simulink model "simulation_3d"  (R2023b)
settings: Solver=ode4  StartTime=0.0  StopTime=2  FixedStep=0.001  RelTol=1e-3  EnableMultiTasking=on
values from neighbouring files (symbols this model uses):
  compKd = 1    [main.m]
  compKi = 0    [main.m]
  compKp = 1    [main.m]
  derivative_filter_samples = 1    [parameters.m]
  gain = 0.00285714285714    [paper_data.mat]    (also in parameters.m = 0.025)
  initial_q = q    [main.m]    (also in paper_data.mat = [0 0 0 0.2 0 0.2]; stuff.mat = [0 0 0 0 0 0])
  initial_states = [tau(1), tau(2), q_dot(1), q_dot(2), q_dot(3), q_dot(4),                     q_dot(5), q_dot(6),q(1), q(2), q(3), q(4), q(5), q(6),                     x_ICR, v(1), v(2), bld_ang(1), bld_ang(2), bld_ang(3)]    [main.m]    (also in paper_data.mat = [56000 56000 0 0 0 0 0 0 0 0 0 0.2 ... (20 elements, 1x20)]; stuff.mat = [56000 56000 0 0 0 0 0 0 0 0 0 0 ... (20 elements, 20x1)])
  initial_v = v    [main.m]    (also in paper_data.mat = [0 0]; stuff.mat = [0 0])
  L = 1.4    [paper_data.mat]    (also in parameters.m = 1.2; stuff.mat)
  l = 2.349    [paper_data.mat]    (also in parameters.m; stuff.mat; test.m = vd_parmas(3))
  stop_distance = 0.3    [paper_data.mat]    (also in parameters.m)
  type = 0.9    [paper_data.mat]    (also in parameters.m; stuff.mat = 0.2)
  v_limit = [velocity_limit, turn_vel_limit]    [main.m]
undefined symbols (not defined in the file or in its folder): DiscIntNeverNeededParam
libraries: fuzblock x10, slpidlib x6, simulink x2
settings Model: Creator=frog  LastModifiedBy=srd2
settings SolverCC: AlgebraicLoopSolver=TrustRegion
settings DataIOCC: ExternalInput=[in]  InitialState=pathlength
settings DebuggingCC: UnconnectedInputMsg=warning  UnconnectedOutputMsg=warning  UnconnectedLineMsg=warning  UnderSpecifiedDimensionMsg=warning
settings ModelReferenceCC: EnableRefExpFcnMdlSchedulingChecks=on
settings RTWCC: DLArmComputeVersion=19.05

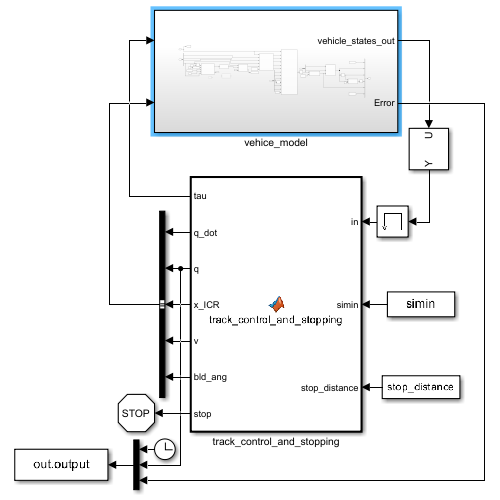
[thumbnail: Simulink's stored preview of the top-level diagram]
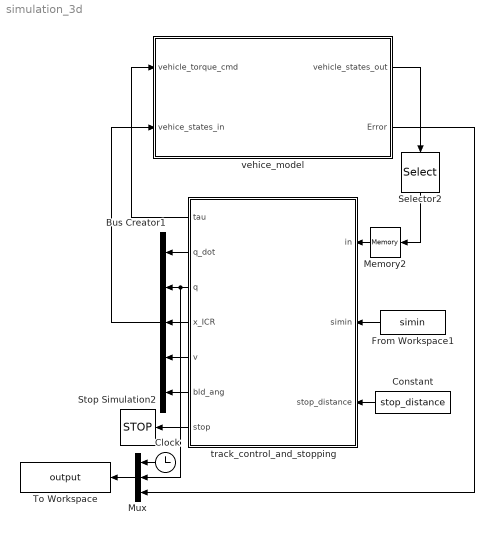
== system simulation_3d ==
  Bus Creator1 : BusCreator  Inputs=5
  Clock : Clock
  Constant : Constant  Value=stop_distance
  From Workspace1 : FromWorkspace  VariableName=simin
  Memory2 : Memory  InitialCondition=initial_states  InheritSampleTime=on
  Mux : Mux  Inputs=3
  Selector2 : Selector  InputPortWidth=20  IndexOptions=Index vector (dialog)  Indices=[1 2 3 4 5 6 7 8 9 10 11 12 13 14 15 16 17 18 19 20]  OutputSizes=1
  Stop Simulation2 : Stop
  To Workspace : ToWorkspace  VariableName=output  SaveFormat=Timeseries  SampleTime=-1
  track_control_and_stopping : MATLAB Function  TreatAsAtomicUnit=on
  vehice_model : Subsystem
  wires:
  Bus Creator1/1 -> vehice_model/2(vehice_states_in)
  vehice_model/1(vehicle_states_out) -> Selector2/1
  track_control_and_stopping/7(stop) -> Stop Simulation2/1
  From Workspace1/1 -> track_control_and_stopping/2(simin)
  Selector2/1 -> Memory2/1
  Memory2/1 -> track_control_and_stopping/1(in)
  track_control_and_stopping/5(v) -> Bus Creator1/4
  track_control_and_stopping/4(x_ICR) -> Bus Creator1/3
  track_control_and_stopping/3(q) -> Bus Creator1/2, Mux/2
  track_control_and_stopping/1(tau) -> vehice_model/1(vehicle_torque_cmd)
  track_control_and_stopping/6(bld_ang) -> Bus Creator1/5
  Mux/1 -> To Workspace/1
  Clock/1 -> Mux/1
  vehice_model/2(Error) -> Mux/3
  Constant/1 -> track_control_and_stopping/3(stop_distance)
  track_control_and_stopping/2(q_dot) -> Bus Creator1/1

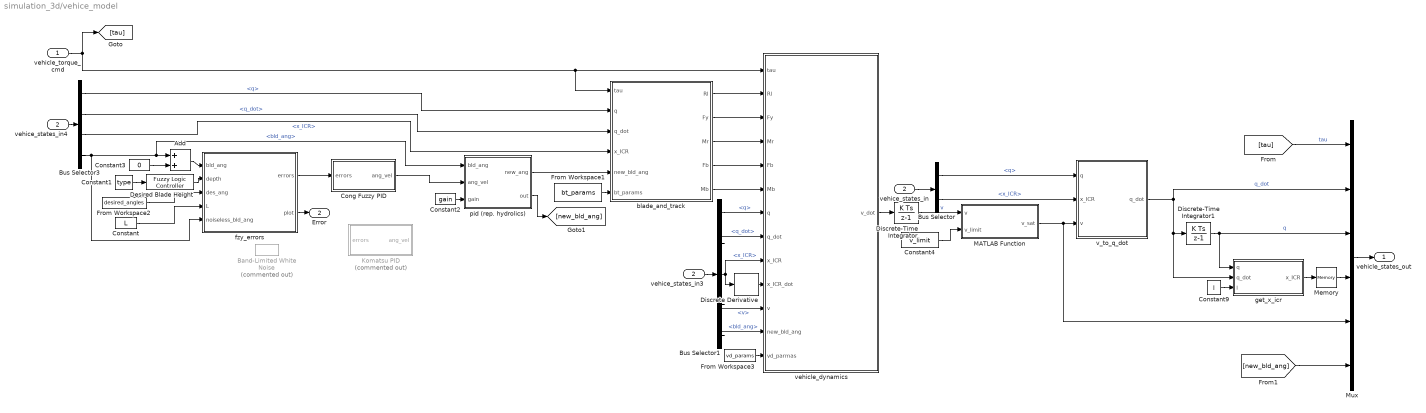
== system simulation_3d/vehice_model ==
  vehicle_torque_cmd : Inport
  vehice_states_in : Inport  Port=2
  Add : Sum
  Band-Limited White Noise : simulink/Sources/Band-Limited White Noise  Commented=on  Cov=[1e-4]  Ts=0.0001  seed=[23341]
  Bus Selector : BusSelector  OutputSignals=q,x_ICR
  Bus Selector1 : BusSelector  OutputSignals=q,q_dot,x_ICR,v,bld_ang
  Bus Selector3 : BusSelector  OutputSignals=q,q_dot,x_ICR,bld_ang
  Cong Fuzzy PID : Subsystem
  Constant : Constant  Value=L
  Constant1 : Constant  Value=type
  Constant2 : Constant  Value=gain
  Constant3 : Constant  Value=0
  Constant4 : Constant  Value=v_limit
  Constant9 : Constant  Value=l
  Desired Blade Height : fuzblock/Fuzzy Logic  Controller  FIS='blade_height.fis'  OutputSampleNumber=101  DataType=double  FuzzifiedInputs=off  RuleFiringStrengths=off  RuleOutputs=off  AggregatedOutputs=off  SimulateUsing=Interpreted execution  OutOfRangeInputValueMessage=warning  NoRuleFiredMessage=warning  EmptyOutputFuzzySetMessage=warning
  Discrete Derivative : simulink/Discrete/Discrete Derivative  gainval=1.0  ICPrevScaledInput=0.0  OutMin=[]  OutMax=[]  OutDataType=fixdt(1, 16)  OutScaling=2^-10  DoSatur=off
  Discrete-Time Integrator : DiscreteIntegrator  InitialCondition=initial_v  SampleTime=-1  ICPrevOutput=DiscIntNeverNeededParam  ICPrevScaledInput=DiscIntNeverNeededParam
  Discrete-Time Integrator1 : DiscreteIntegrator  InitialCondition=initial_q  SampleTime=-1  ICPrevOutput=DiscIntNeverNeededParam  ICPrevScaledInput=DiscIntNeverNeededParam
  From Workspace1 : FromWorkspace  VariableName=bt_params
  From Workspace2 : FromWorkspace  VariableName=desired_angles
  From Workspace3 : FromWorkspace  VariableName=vd_params
  Komatsu PID : Subsystem  Commented=on
  MATLAB Function : MATLAB Function  TreatAsAtomicUnit=on
  Memory : Memory  InheritSampleTime=on  LinearizeAsDelay=on
  Mux : Mux  Inputs=6
  blade_and_track : MATLAB Function  TreatAsAtomicUnit=on
  fzy_errors : MATLAB Function  TreatAsAtomicUnit=on
  get_x_icr : MATLAB Function  TreatAsAtomicUnit=on
  pid (rep. hydrolics) : MATLAB Function  TreatAsAtomicUnit=on
  v_to_q_dot : MATLAB Function  TreatAsAtomicUnit=on
  vehice_states_in3 : InportShadow  Port=2
  vehice_states_in4 : InportShadow  Port=2
  vehicle_dynamics : MATLAB Function  TreatAsAtomicUnit=on
  vehicle_states_out : Outport
  Error : Outport  Port=2
  wires:
  Mux/1 -> vehicle_states_out/1
  Discrete-Time Integrator1/1 -> Mux/3, get_x_icr/1(q)  "q"
  v_to_q_dot/1(q_dot) -> Mux/2, Discrete-Time Integrator1/1, get_x_icr/2(q_dot)  "q_dot"
  vehice_states_in/1 -> Bus Selector/1
  vehicle_dynamics/1(v_dot) -> Discrete-Time Integrator/1
  [tau] -> Mux/1  "tau"
  blade_and_track/3(Mr) -> vehicle_dynamics/4(Mr)
  blade_and_track/2(Fy) -> vehicle_dynamics/3(Fy)
  blade_and_track/1(Rl) -> vehicle_dynamics/2(Rl)
  vehice_states_in3/1 -> Bus Selector1/1
  Bus Selector1/2 -> vehicle_dynamics/8(q_dot)  "<q_dot>"
  vehicle_torque_cmd/1 -> blade_and_track/1(tau), vehicle_dynamics/1(tau), [tau]
  Bus Selector3/1 -> blade_and_track/2(q)  "<q>"
  Bus Selector3/2 -> blade_and_track/3(q_dot)  "<q_dot>"
  Bus Selector3/3 -> blade_and_track/4(x_ICR)  "<x_ICR>"
  Bus Selector1/4 -> vehicle_dynamics/11(v)  "<v>"
  Bus Selector/1 -> v_to_q_dot/1(q)  "<q>"
  Bus Selector1/1 -> vehicle_dynamics/7(q)  "<q>"
  Discrete Derivative/1 -> vehicle_dynamics/10(x_ICR_dot)
  Bus Selector1/3 -> vehicle_dynamics/9(x_ICR), Discrete Derivative/1  "<x_ICR>"
  Bus Selector/2 -> v_to_q_dot/2(x_ICR)  "<x_ICR>"
  vehice_states_in4/1 -> Bus Selector3/1
  get_x_icr/1(x_ICR) -> Memory/1
  blade_and_track/4(Fb) -> vehicle_dynamics/5(Fb)
  Desired Blade Height/1 -> fzy_errors/2(depth)
  Bus Selector1/5 -> vehicle_dynamics/12(new_bld_ang)  "<bld_ang>"
  blade_and_track/5(Mb) -> vehicle_dynamics/6(Mb)
  Constant1/1 -> Desired Blade Height/1
  Bus Selector3/4 -> pid (rep. hydrolics)/1(bld_ang), Add/1, fzy_errors/5(noiseless_bld_ang)  "<bld_ang>"
  pid (rep. hydrolics)/1(new_ang) -> blade_and_track/5(new_bld_ang)
  [new_bld_ang] -> Mux/6
  pid (rep. hydrolics)/2(out) -> [new_bld_ang]
  Constant9/1 -> get_x_icr/3(l)
  From Workspace2/1 -> fzy_errors/3(des_ang)
  From Workspace1/1 -> blade_and_track/6(bt_params)
  From Workspace3/1 -> vehicle_dynamics/13(vd_parmas)
  fzy_errors/2(plot) -> Error/1
  Constant/1 -> fzy_errors/4(L)
  Constant2/1 -> pid (rep. hydrolics)/3(gain)
  Memory/1 -> Mux/4
  Add/1 -> fzy_errors/1(bld_ang)
  Constant3/1 -> Add/2
  Constant4/1 -> MATLAB Function/2(v_limit)
  Discrete-Time Integrator/1 -> MATLAB Function/1(v)  "v"
  MATLAB Function/1(v_sat) -> v_to_q_dot/3(v), Mux/5
  fzy_errors/1(errors) -> Cong Fuzzy PID/1(errors)
  Cong Fuzzy PID/1(ang_vel) -> pid (rep. hydrolics)/2(ang_vel)

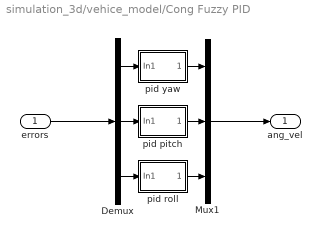
== system simulation_3d/vehice_model/Cong Fuzzy PID ==
  errors : Inport
  Demux : Demux  Outputs=3
  Mux1 : Mux  Inputs=3
  pid pitch : Subsystem
  pid roll : Subsystem
  pid yaw : Subsystem
  ang_vel : Outport
  wires:
  Demux/2 -> pid pitch/1(In1)
  pid yaw/1(Out1) -> Mux1/1
  Demux/3 -> pid roll/1(In1)
  pid roll/1(Out1) -> Mux1/3
  pid pitch/1(Out1) -> Mux1/2
  Demux/1 -> pid yaw/1(In1)
  errors/1 -> Demux/1
  Mux1/1 -> ang_vel/1

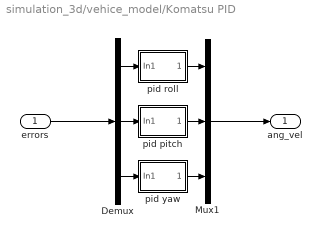
== system simulation_3d/vehice_model/Komatsu PID ==
  errors : Inport
  Demux : Demux  Outputs=3
  Mux1 : Mux  Inputs=3
  pid pitch : Subsystem
  pid roll : Subsystem
  pid yaw : Subsystem
  ang_vel : Outport
  wires:
  Demux/2 -> pid pitch/1(In1)
  pid roll/1(Out1) -> Mux1/1
  Demux/3 -> pid yaw/1(In1)
  pid yaw/1(Out1) -> Mux1/3
  pid pitch/1(Out1) -> Mux1/2
  Demux/1 -> pid roll/1(In1)
  errors/1 -> Demux/1
  Mux1/1 -> ang_vel/1

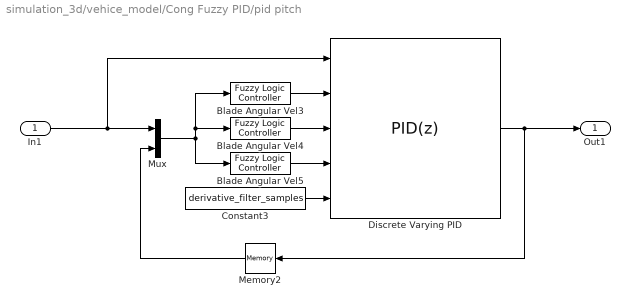
== system simulation_3d/vehice_model/Cong Fuzzy PID/pid pitch ==
  In1 : Inport
  Blade Angular Vel3 : fuzblock/Fuzzy Logic  Controller  FIS='comparision_Kp.fis'  OutputSampleNumber=101  DataType=double  FuzzifiedInputs=off  RuleFiringStrengths=off  RuleOutputs=off  AggregatedOutputs=off  SimulateUsing=Interpreted execution  OutOfRangeInputValueMessage=warning  NoRuleFiredMessage=warning  EmptyOutputFuzzySetMessage=warning
  Blade Angular Vel4 : fuzblock/Fuzzy Logic  Controller  FIS='comparision_Ki.fis'  OutputSampleNumber=101  DataType=double  FuzzifiedInputs=off  RuleFiringStrengths=off  RuleOutputs=off  AggregatedOutputs=off  SimulateUsing=Interpreted execution  OutOfRangeInputValueMessage=warning  NoRuleFiredMessage=warning  EmptyOutputFuzzySetMessage=warning
  Blade Angular Vel5 : fuzblock/Fuzzy Logic  Controller  FIS='comparision_Kd.fis'  OutputSampleNumber=101  DataType=double  FuzzifiedInputs=off  RuleFiringStrengths=off  RuleOutputs=off  AggregatedOutputs=off  SimulateUsing=Interpreted execution  OutOfRangeInputValueMessage=warning  NoRuleFiredMessage=warning  EmptyOutputFuzzySetMessage=warning
  Constant3 : Constant  Value=derivative_filter_samples
  Discrete Varying PID : slpidlib/PID Controller  Controller=PID  Form=Parallel  TimeDomain=Discrete-time  UseExternalTs=off  SampleTime=-1  IntegratorMethod=Forward Euler  FilterMethod=Forward Euler  ControllerParametersSource=external  P=1  I=1  UseKiTs=off  D=0  N=100  UseFilter=on  TunerSelectOption=Transfer Function Based (PID Tuner App)  InitialConditionSource=internal  InitialConditionForIntegrator=0  InitialConditionForFilter=0  DifferentiatorICPrevScaledInput=0  ExternalReset=none  TrackingMode=off  Kt=1  LimitOutput=off  SatLimitsSource=internal  UpperSaturationLimit=inf  LowerSaturationLimit=-inf  LinearizeAsGain=on  AntiWindupMode=none  Kb=1  LimitIntegrator=off  UpperIntegratorSaturationLimit=inf  LowerIntegratorSaturationLimit=-inf  POutMin=[]  POutMax=[]  IOutMin=[]  IOutMax=[]  DOutMin=[]  DOutMax=[]  NOutMin=[]  NOutMax=[]  SumOutMin=[]  SumOutMax=[]  SaturationOutMin=[]  SaturationOutMax=[]  PParamMin=[]  PParamMax=[]  IParamMin=[]  IParamMax=[]  DParamMin=[]  DParamMax=[]  NParamMin=[]  NParamMax=[]  KbParamMin=[]  KbParamMax=[]  KtParamMin=[]  KtParamMax=[]  KbOutMin=[]  KbOutMax=[]  KtOutMin=[]  KtOutMax=[]  IntegratorOutMin=[]  IntegratorOutMax=[]  FilterOutMin=[]  FilterOutMax=[]  SumI1OutMin=[]  SumI1OutMax=[]  SumI2OutMin=[]  SumI2OutMax=[]  SumI3OutMin=[]  SumI3OutMax=[]  SumI4OutMin=[]  SumI4OutMax=[]  SumDOutMin=[]  SumDOutMax=[]  DifferentiatorOutMin=[]  DifferentiatorOutMax=[]  FilterDiffOutCoefMin=[]  FilterDiffOutCoefMax=[]  ReciprocalOutMin=[]  ReciprocalOutMax=[]  SumDenOutMin=[]  SumDenOutMax=[]  SumNumOutMin=[]  SumNumOutMax=[]  DivideOutMin=[]  DivideOutMax=[]  UdiffTsProdOutMin=[]  UdiffTsProdOutMax=[]  NTsProdOutMin=[]  NTsProdOutMax=[]  UintegralTsProdOutMin=[]  UintegralTsProdOutMax=[]  UngainTsProdOutMin=[]  UngainTsProdOutMax=[]  ClampingZeroOutDataTypeStr=Inherit: Inherit via back propagation  ClampingZeroOutMin=[]  ClampingZeroOutMax=[]  FilterDenConstantOutDataTypeStr=Inherit: Inherit via back propagation  FilterDenConstantOutMin=[]  FilterDenConstantOutMax=[]  PCopyOutDataTypeStr=Inherit: Inherit via back propagation  PCopyOutMin=[]  PCopyOutMax=[]  NCopyOutDataTypeStr=Inherit: Inherit via back propagation  NCopyOutMin=[]  NCopyOutMax=[]  IntegratorContinuousStateAttributes=''  IntegratorStateMustResolveToSignalObject=off  IntegratorRTWStateStorageClass=Auto  FilterContinuousStateAttributes=''  FilterStateMustResolveToSignalObject=off  FilterRTWStateStorageClass=Auto  ParallelPVariant=ExternalParameters  IdealPVariant=Disabled  IVariant=ExternalParameters  DVariant=ExternalParameters  IntegratorVariant=Discrete  SatVariant=Disabled  AWVariant=Passthrough  PCopyVariant=Disabled  TRVariant=Disabled  FdbkBlocksVariant=Forward  IdealPFdbkVariant=Disabled  SatFdbkVariant=Disabled  DerivativeFilterVariant=ForwardEulerFilter  NVariant=ExternalParameters  NCopyVariant=Disabled  FilterICVariant=InternalICsFilter  IntegratorICVariant=InternalICs  ExternalResetVariant=Disabled  TRSumVariant=Passthrough  SumFdbkVariant=Disabled  SumVariant=Sum_PID  TsampFilterVariant=InternalTs  TsampNgainVariant=Passthrough  TsampIntegralVariant=Disabled_SignalSpec  ExternalSaturationOutDataTypeStr=Inherit: Same as second input
      settings: LibrarySourceBlock=cstblocks/Linear Parameter Varying/Discrete Varying PID
  Memory2 : Memory  InheritSampleTime=on  LinearizeAsDelay=on
  Mux : Mux  Inputs=2
  Out1 : Outport
  wires:
  Blade Angular Vel5/1 -> Discrete Varying PID/4
  Discrete Varying PID/1 -> Memory2/1, Out1/1
  Constant3/1 -> Discrete Varying PID/5
  Blade Angular Vel3/1 -> Discrete Varying PID/2
  Blade Angular Vel4/1 -> Discrete Varying PID/3
  In1/1 -> Mux/1, Discrete Varying PID/1
  Memory2/1 -> Mux/2
  Mux/1 -> Blade Angular Vel5/1, Blade Angular Vel4/1, Blade Angular Vel3/1

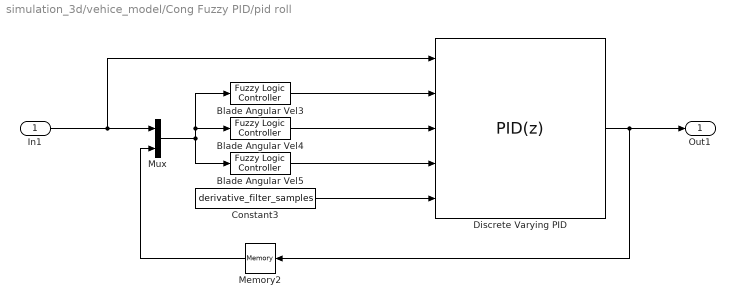
== system simulation_3d/vehice_model/Cong Fuzzy PID/pid roll ==
  In1 : Inport
  Blade Angular Vel3 : fuzblock/Fuzzy Logic  Controller  FIS='comparision_Kp.fis'  OutputSampleNumber=101  DataType=double  FuzzifiedInputs=off  RuleFiringStrengths=off  RuleOutputs=off  AggregatedOutputs=off  SimulateUsing=Interpreted execution  OutOfRangeInputValueMessage=warning  NoRuleFiredMessage=warning  EmptyOutputFuzzySetMessage=warning
  Blade Angular Vel4 : fuzblock/Fuzzy Logic  Controller  FIS='comparision_Ki.fis'  OutputSampleNumber=101  DataType=double  FuzzifiedInputs=off  RuleFiringStrengths=off  RuleOutputs=off  AggregatedOutputs=off  SimulateUsing=Interpreted execution  OutOfRangeInputValueMessage=warning  NoRuleFiredMessage=warning  EmptyOutputFuzzySetMessage=warning
  Blade Angular Vel5 : fuzblock/Fuzzy Logic  Controller  FIS='comparision_Kd.fis'  OutputSampleNumber=101  DataType=double  FuzzifiedInputs=off  RuleFiringStrengths=off  RuleOutputs=off  AggregatedOutputs=off  SimulateUsing=Interpreted execution  OutOfRangeInputValueMessage=warning  NoRuleFiredMessage=warning  EmptyOutputFuzzySetMessage=warning
  Constant3 : Constant  Value=derivative_filter_samples
  Discrete Varying PID : slpidlib/PID Controller  Controller=PID  Form=Parallel  TimeDomain=Discrete-time  UseExternalTs=off  SampleTime=-1  IntegratorMethod=Forward Euler  FilterMethod=Forward Euler  ControllerParametersSource=external  P=1  I=1  UseKiTs=off  D=0  N=100  UseFilter=on  TunerSelectOption=Transfer Function Based (PID Tuner App)  InitialConditionSource=internal  InitialConditionForIntegrator=0  InitialConditionForFilter=0  DifferentiatorICPrevScaledInput=0  ExternalReset=none  TrackingMode=off  Kt=1  LimitOutput=off  SatLimitsSource=internal  UpperSaturationLimit=inf  LowerSaturationLimit=-inf  LinearizeAsGain=on  AntiWindupMode=none  Kb=1  LimitIntegrator=off  UpperIntegratorSaturationLimit=inf  LowerIntegratorSaturationLimit=-inf  POutMin=[]  POutMax=[]  IOutMin=[]  IOutMax=[]  DOutMin=[]  DOutMax=[]  NOutMin=[]  NOutMax=[]  SumOutMin=[]  SumOutMax=[]  SaturationOutMin=[]  SaturationOutMax=[]  PParamMin=[]  PParamMax=[]  IParamMin=[]  IParamMax=[]  DParamMin=[]  DParamMax=[]  NParamMin=[]  NParamMax=[]  KbParamMin=[]  KbParamMax=[]  KtParamMin=[]  KtParamMax=[]  KbOutMin=[]  KbOutMax=[]  KtOutMin=[]  KtOutMax=[]  IntegratorOutMin=[]  IntegratorOutMax=[]  FilterOutMin=[]  FilterOutMax=[]  SumI1OutMin=[]  SumI1OutMax=[]  SumI2OutMin=[]  SumI2OutMax=[]  SumI3OutMin=[]  SumI3OutMax=[]  SumI4OutMin=[]  SumI4OutMax=[]  SumDOutMin=[]  SumDOutMax=[]  DifferentiatorOutMin=[]  DifferentiatorOutMax=[]  FilterDiffOutCoefMin=[]  FilterDiffOutCoefMax=[]  ReciprocalOutMin=[]  ReciprocalOutMax=[]  SumDenOutMin=[]  SumDenOutMax=[]  SumNumOutMin=[]  SumNumOutMax=[]  DivideOutMin=[]  DivideOutMax=[]  UdiffTsProdOutMin=[]  UdiffTsProdOutMax=[]  NTsProdOutMin=[]  NTsProdOutMax=[]  UintegralTsProdOutMin=[]  UintegralTsProdOutMax=[]  UngainTsProdOutMin=[]  UngainTsProdOutMax=[]  ClampingZeroOutDataTypeStr=Inherit: Inherit via back propagation  ClampingZeroOutMin=[]  ClampingZeroOutMax=[]  FilterDenConstantOutDataTypeStr=Inherit: Inherit via back propagation  FilterDenConstantOutMin=[]  FilterDenConstantOutMax=[]  PCopyOutDataTypeStr=Inherit: Inherit via back propagation  PCopyOutMin=[]  PCopyOutMax=[]  NCopyOutDataTypeStr=Inherit: Inherit via back propagation  NCopyOutMin=[]  NCopyOutMax=[]  IntegratorContinuousStateAttributes=''  IntegratorStateMustResolveToSignalObject=off  IntegratorRTWStateStorageClass=Auto  FilterContinuousStateAttributes=''  FilterStateMustResolveToSignalObject=off  FilterRTWStateStorageClass=Auto  ParallelPVariant=ExternalParameters  IdealPVariant=Disabled  IVariant=ExternalParameters  DVariant=ExternalParameters  IntegratorVariant=Discrete  SatVariant=Disabled  AWVariant=Passthrough  PCopyVariant=Disabled  TRVariant=Disabled  FdbkBlocksVariant=Forward  IdealPFdbkVariant=Disabled  SatFdbkVariant=Disabled  DerivativeFilterVariant=ForwardEulerFilter  NVariant=ExternalParameters  NCopyVariant=Disabled  FilterICVariant=InternalICsFilter  IntegratorICVariant=InternalICs  ExternalResetVariant=Disabled  TRSumVariant=Passthrough  SumFdbkVariant=Disabled  SumVariant=Sum_PID  TsampFilterVariant=InternalTs  TsampNgainVariant=Passthrough  TsampIntegralVariant=Disabled_SignalSpec  ExternalSaturationOutDataTypeStr=Inherit: Same as second input
      settings: LibrarySourceBlock=cstblocks/Linear Parameter Varying/Discrete Varying PID
  Memory2 : Memory  InheritSampleTime=on  LinearizeAsDelay=on
  Mux : Mux  Inputs=2
  Out1 : Outport
  wires:
  Blade Angular Vel5/1 -> Discrete Varying PID/4
  Discrete Varying PID/1 -> Memory2/1, Out1/1
  Constant3/1 -> Discrete Varying PID/5
  Blade Angular Vel3/1 -> Discrete Varying PID/2
  Blade Angular Vel4/1 -> Discrete Varying PID/3
  In1/1 -> Mux/1, Discrete Varying PID/1
  Memory2/1 -> Mux/2
  Mux/1 -> Blade Angular Vel5/1, Blade Angular Vel4/1, Blade Angular Vel3/1

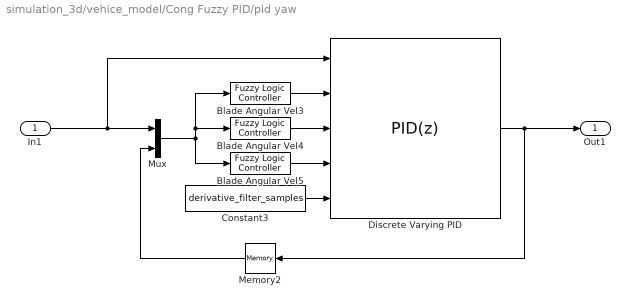
== system simulation_3d/vehice_model/Cong Fuzzy PID/pid yaw ==
  In1 : Inport
  Blade Angular Vel3 : fuzblock/Fuzzy Logic  Controller  FIS='comparision_Kp.fis'  OutputSampleNumber=101  DataType=double  FuzzifiedInputs=off  RuleFiringStrengths=off  RuleOutputs=off  AggregatedOutputs=off  SimulateUsing=Interpreted execution  OutOfRangeInputValueMessage=warning  NoRuleFiredMessage=warning  EmptyOutputFuzzySetMessage=warning
  Blade Angular Vel4 : fuzblock/Fuzzy Logic  Controller  FIS='comparision_Ki.fis'  OutputSampleNumber=101  DataType=double  FuzzifiedInputs=off  RuleFiringStrengths=off  RuleOutputs=off  AggregatedOutputs=off  SimulateUsing=Interpreted execution  OutOfRangeInputValueMessage=warning  NoRuleFiredMessage=warning  EmptyOutputFuzzySetMessage=warning
  Blade Angular Vel5 : fuzblock/Fuzzy Logic  Controller  FIS='comparision_Kd.fis'  OutputSampleNumber=101  DataType=double  FuzzifiedInputs=off  RuleFiringStrengths=off  RuleOutputs=off  AggregatedOutputs=off  SimulateUsing=Interpreted execution  OutOfRangeInputValueMessage=warning  NoRuleFiredMessage=warning  EmptyOutputFuzzySetMessage=warning
  Constant3 : Constant  Value=derivative_filter_samples
  Discrete Varying PID : slpidlib/PID Controller  Controller=PID  Form=Parallel  TimeDomain=Discrete-time  UseExternalTs=off  SampleTime=-1  IntegratorMethod=Forward Euler  FilterMethod=Forward Euler  ControllerParametersSource=external  P=1  I=1  UseKiTs=off  D=0  N=100  UseFilter=on  TunerSelectOption=Transfer Function Based (PID Tuner App)  InitialConditionSource=internal  InitialConditionForIntegrator=0  InitialConditionForFilter=0  DifferentiatorICPrevScaledInput=0  ExternalReset=none  TrackingMode=off  Kt=1  LimitOutput=off  SatLimitsSource=internal  UpperSaturationLimit=inf  LowerSaturationLimit=-inf  LinearizeAsGain=on  AntiWindupMode=none  Kb=1  LimitIntegrator=off  UpperIntegratorSaturationLimit=inf  LowerIntegratorSaturationLimit=-inf  POutMin=[]  POutMax=[]  IOutMin=[]  IOutMax=[]  DOutMin=[]  DOutMax=[]  NOutMin=[]  NOutMax=[]  SumOutMin=[]  SumOutMax=[]  SaturationOutMin=[]  SaturationOutMax=[]  PParamMin=[]  PParamMax=[]  IParamMin=[]  IParamMax=[]  DParamMin=[]  DParamMax=[]  NParamMin=[]  NParamMax=[]  KbParamMin=[]  KbParamMax=[]  KtParamMin=[]  KtParamMax=[]  KbOutMin=[]  KbOutMax=[]  KtOutMin=[]  KtOutMax=[]  IntegratorOutMin=[]  IntegratorOutMax=[]  FilterOutMin=[]  FilterOutMax=[]  SumI1OutMin=[]  SumI1OutMax=[]  SumI2OutMin=[]  SumI2OutMax=[]  SumI3OutMin=[]  SumI3OutMax=[]  SumI4OutMin=[]  SumI4OutMax=[]  SumDOutMin=[]  SumDOutMax=[]  DifferentiatorOutMin=[]  DifferentiatorOutMax=[]  FilterDiffOutCoefMin=[]  FilterDiffOutCoefMax=[]  ReciprocalOutMin=[]  ReciprocalOutMax=[]  SumDenOutMin=[]  SumDenOutMax=[]  SumNumOutMin=[]  SumNumOutMax=[]  DivideOutMin=[]  DivideOutMax=[]  UdiffTsProdOutMin=[]  UdiffTsProdOutMax=[]  NTsProdOutMin=[]  NTsProdOutMax=[]  UintegralTsProdOutMin=[]  UintegralTsProdOutMax=[]  UngainTsProdOutMin=[]  UngainTsProdOutMax=[]  ClampingZeroOutDataTypeStr=Inherit: Inherit via back propagation  ClampingZeroOutMin=[]  ClampingZeroOutMax=[]  FilterDenConstantOutDataTypeStr=Inherit: Inherit via back propagation  FilterDenConstantOutMin=[]  FilterDenConstantOutMax=[]  PCopyOutDataTypeStr=Inherit: Inherit via back propagation  PCopyOutMin=[]  PCopyOutMax=[]  NCopyOutDataTypeStr=Inherit: Inherit via back propagation  NCopyOutMin=[]  NCopyOutMax=[]  IntegratorContinuousStateAttributes=''  IntegratorStateMustResolveToSignalObject=off  IntegratorRTWStateStorageClass=Auto  FilterContinuousStateAttributes=''  FilterStateMustResolveToSignalObject=off  FilterRTWStateStorageClass=Auto  ParallelPVariant=ExternalParameters  IdealPVariant=Disabled  IVariant=ExternalParameters  DVariant=ExternalParameters  IntegratorVariant=Discrete  SatVariant=Disabled  AWVariant=Passthrough  PCopyVariant=Disabled  TRVariant=Disabled  FdbkBlocksVariant=Forward  IdealPFdbkVariant=Disabled  SatFdbkVariant=Disabled  DerivativeFilterVariant=ForwardEulerFilter  NVariant=ExternalParameters  NCopyVariant=Disabled  FilterICVariant=InternalICsFilter  IntegratorICVariant=InternalICs  ExternalResetVariant=Disabled  TRSumVariant=Passthrough  SumFdbkVariant=Disabled  SumVariant=Sum_PID  TsampFilterVariant=InternalTs  TsampNgainVariant=Passthrough  TsampIntegralVariant=Disabled_SignalSpec  ExternalSaturationOutDataTypeStr=Inherit: Same as second input
      settings: LibrarySourceBlock=cstblocks/Linear Parameter Varying/Discrete Varying PID
  Memory2 : Memory  InheritSampleTime=on  LinearizeAsDelay=on
  Mux : Mux  Inputs=2
  Out1 : Outport
  wires:
  Blade Angular Vel5/1 -> Discrete Varying PID/4
  Discrete Varying PID/1 -> Memory2/1, Out1/1
  Constant3/1 -> Discrete Varying PID/5
  Blade Angular Vel3/1 -> Discrete Varying PID/2
  Blade Angular Vel4/1 -> Discrete Varying PID/3
  In1/1 -> Mux/1, Discrete Varying PID/1
  Memory2/1 -> Mux/2
  Mux/1 -> Blade Angular Vel5/1, Blade Angular Vel4/1, Blade Angular Vel3/1

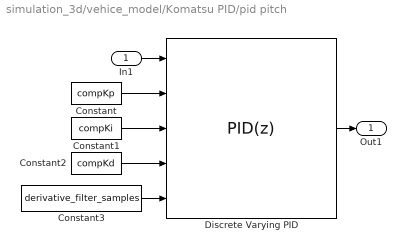
== system simulation_3d/vehice_model/Komatsu PID/pid pitch ==
  In1 : Inport
  Constant : Constant  Value=compKp
  Constant1 : Constant  Value=compKi
  Constant2 : Constant  Value=compKd
  Constant3 : Constant  Value=derivative_filter_samples
  Discrete Varying PID : slpidlib/PID Controller  Controller=PID  Form=Parallel  TimeDomain=Discrete-time  UseExternalTs=off  SampleTime=-1  IntegratorMethod=Forward Euler  FilterMethod=Forward Euler  ControllerParametersSource=external  P=1  I=1  UseKiTs=off  D=0  N=100  UseFilter=on  TunerSelectOption=Transfer Function Based (PID Tuner App)  InitialConditionSource=internal  InitialConditionForIntegrator=0  InitialConditionForFilter=0  DifferentiatorICPrevScaledInput=0  ExternalReset=none  TrackingMode=off  Kt=1  LimitOutput=off  SatLimitsSource=internal  UpperSaturationLimit=inf  LowerSaturationLimit=-inf  LinearizeAsGain=on  AntiWindupMode=none  Kb=1  LimitIntegrator=off  UpperIntegratorSaturationLimit=inf  LowerIntegratorSaturationLimit=-inf  POutMin=[]  POutMax=[]  IOutMin=[]  IOutMax=[]  DOutMin=[]  DOutMax=[]  NOutMin=[]  NOutMax=[]  SumOutMin=[]  SumOutMax=[]  SaturationOutMin=[]  SaturationOutMax=[]  PParamMin=[]  PParamMax=[]  IParamMin=[]  IParamMax=[]  DParamMin=[]  DParamMax=[]  NParamMin=[]  NParamMax=[]  KbParamMin=[]  KbParamMax=[]  KtParamMin=[]  KtParamMax=[]  KbOutMin=[]  KbOutMax=[]  KtOutMin=[]  KtOutMax=[]  IntegratorOutMin=[]  IntegratorOutMax=[]  FilterOutMin=[]  FilterOutMax=[]  SumI1OutMin=[]  SumI1OutMax=[]  SumI2OutMin=[]  SumI2OutMax=[]  SumI3OutMin=[]  SumI3OutMax=[]  SumI4OutMin=[]  SumI4OutMax=[]  SumDOutMin=[]  SumDOutMax=[]  DifferentiatorOutMin=[]  DifferentiatorOutMax=[]  FilterDiffOutCoefMin=[]  FilterDiffOutCoefMax=[]  ReciprocalOutMin=[]  ReciprocalOutMax=[]  SumDenOutMin=[]  SumDenOutMax=[]  SumNumOutMin=[]  SumNumOutMax=[]  DivideOutMin=[]  DivideOutMax=[]  UdiffTsProdOutMin=[]  UdiffTsProdOutMax=[]  NTsProdOutMin=[]  NTsProdOutMax=[]  UintegralTsProdOutMin=[]  UintegralTsProdOutMax=[]  UngainTsProdOutMin=[]  UngainTsProdOutMax=[]  ClampingZeroOutDataTypeStr=Inherit: Inherit via back propagation  ClampingZeroOutMin=[]  ClampingZeroOutMax=[]  FilterDenConstantOutDataTypeStr=Inherit: Inherit via back propagation  FilterDenConstantOutMin=[]  FilterDenConstantOutMax=[]  PCopyOutDataTypeStr=Inherit: Inherit via back propagation  PCopyOutMin=[]  PCopyOutMax=[]  NCopyOutDataTypeStr=Inherit: Inherit via back propagation  NCopyOutMin=[]  NCopyOutMax=[]  IntegratorContinuousStateAttributes=''  IntegratorStateMustResolveToSignalObject=off  IntegratorRTWStateStorageClass=Auto  FilterContinuousStateAttributes=''  FilterStateMustResolveToSignalObject=off  FilterRTWStateStorageClass=Auto  ParallelPVariant=ExternalParameters  IdealPVariant=Disabled  IVariant=ExternalParameters  DVariant=ExternalParameters  IntegratorVariant=Discrete  SatVariant=Disabled  AWVariant=Passthrough  PCopyVariant=Disabled  TRVariant=Disabled  FdbkBlocksVariant=Forward  IdealPFdbkVariant=Disabled  SatFdbkVariant=Disabled  DerivativeFilterVariant=ForwardEulerFilter  NVariant=ExternalParameters  NCopyVariant=Disabled  FilterICVariant=InternalICsFilter  IntegratorICVariant=InternalICs  ExternalResetVariant=Disabled  TRSumVariant=Passthrough  SumFdbkVariant=Disabled  SumVariant=Sum_PID  TsampFilterVariant=InternalTs  TsampNgainVariant=Passthrough  TsampIntegralVariant=Disabled_SignalSpec  ExternalSaturationOutDataTypeStr=Inherit: Same as second input
      settings: LibrarySourceBlock=cstblocks/Linear Parameter Varying/Discrete Varying PID
  Out1 : Outport
  wires:
  Constant2/1 -> Discrete Varying PID/4
  Discrete Varying PID/1 -> Out1/1
  Constant3/1 -> Discrete Varying PID/5
  Constant/1 -> Discrete Varying PID/2
  Constant1/1 -> Discrete Varying PID/3
  In1/1 -> Discrete Varying PID/1

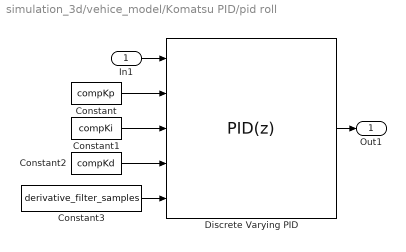
== system simulation_3d/vehice_model/Komatsu PID/pid roll ==
  In1 : Inport
  Constant : Constant  Value=compKp
  Constant1 : Constant  Value=compKi
  Constant2 : Constant  Value=compKd
  Constant3 : Constant  Value=derivative_filter_samples
  Discrete Varying PID : slpidlib/PID Controller  Controller=PID  Form=Parallel  TimeDomain=Discrete-time  UseExternalTs=off  SampleTime=-1  IntegratorMethod=Forward Euler  FilterMethod=Forward Euler  ControllerParametersSource=external  P=1  I=1  UseKiTs=off  D=0  N=100  UseFilter=on  TunerSelectOption=Transfer Function Based (PID Tuner App)  InitialConditionSource=internal  InitialConditionForIntegrator=0  InitialConditionForFilter=0  DifferentiatorICPrevScaledInput=0  ExternalReset=none  TrackingMode=off  Kt=1  LimitOutput=off  SatLimitsSource=internal  UpperSaturationLimit=inf  LowerSaturationLimit=-inf  LinearizeAsGain=on  AntiWindupMode=none  Kb=1  LimitIntegrator=off  UpperIntegratorSaturationLimit=inf  LowerIntegratorSaturationLimit=-inf  POutMin=[]  POutMax=[]  IOutMin=[]  IOutMax=[]  DOutMin=[]  DOutMax=[]  NOutMin=[]  NOutMax=[]  SumOutMin=[]  SumOutMax=[]  SaturationOutMin=[]  SaturationOutMax=[]  PParamMin=[]  PParamMax=[]  IParamMin=[]  IParamMax=[]  DParamMin=[]  DParamMax=[]  NParamMin=[]  NParamMax=[]  KbParamMin=[]  KbParamMax=[]  KtParamMin=[]  KtParamMax=[]  KbOutMin=[]  KbOutMax=[]  KtOutMin=[]  KtOutMax=[]  IntegratorOutMin=[]  IntegratorOutMax=[]  FilterOutMin=[]  FilterOutMax=[]  SumI1OutMin=[]  SumI1OutMax=[]  SumI2OutMin=[]  SumI2OutMax=[]  SumI3OutMin=[]  SumI3OutMax=[]  SumI4OutMin=[]  SumI4OutMax=[]  SumDOutMin=[]  SumDOutMax=[]  DifferentiatorOutMin=[]  DifferentiatorOutMax=[]  FilterDiffOutCoefMin=[]  FilterDiffOutCoefMax=[]  ReciprocalOutMin=[]  ReciprocalOutMax=[]  SumDenOutMin=[]  SumDenOutMax=[]  SumNumOutMin=[]  SumNumOutMax=[]  DivideOutMin=[]  DivideOutMax=[]  UdiffTsProdOutMin=[]  UdiffTsProdOutMax=[]  NTsProdOutMin=[]  NTsProdOutMax=[]  UintegralTsProdOutMin=[]  UintegralTsProdOutMax=[]  UngainTsProdOutMin=[]  UngainTsProdOutMax=[]  ClampingZeroOutDataTypeStr=Inherit: Inherit via back propagation  ClampingZeroOutMin=[]  ClampingZeroOutMax=[]  FilterDenConstantOutDataTypeStr=Inherit: Inherit via back propagation  FilterDenConstantOutMin=[]  FilterDenConstantOutMax=[]  PCopyOutDataTypeStr=Inherit: Inherit via back propagation  PCopyOutMin=[]  PCopyOutMax=[]  NCopyOutDataTypeStr=Inherit: Inherit via back propagation  NCopyOutMin=[]  NCopyOutMax=[]  IntegratorContinuousStateAttributes=''  IntegratorStateMustResolveToSignalObject=off  IntegratorRTWStateStorageClass=Auto  FilterContinuousStateAttributes=''  FilterStateMustResolveToSignalObject=off  FilterRTWStateStorageClass=Auto  ParallelPVariant=ExternalParameters  IdealPVariant=Disabled  IVariant=ExternalParameters  DVariant=ExternalParameters  IntegratorVariant=Discrete  SatVariant=Disabled  AWVariant=Passthrough  PCopyVariant=Disabled  TRVariant=Disabled  FdbkBlocksVariant=Forward  IdealPFdbkVariant=Disabled  SatFdbkVariant=Disabled  DerivativeFilterVariant=ForwardEulerFilter  NVariant=ExternalParameters  NCopyVariant=Disabled  FilterICVariant=InternalICsFilter  IntegratorICVariant=InternalICs  ExternalResetVariant=Disabled  TRSumVariant=Passthrough  SumFdbkVariant=Disabled  SumVariant=Sum_PID  TsampFilterVariant=InternalTs  TsampNgainVariant=Passthrough  TsampIntegralVariant=Disabled_SignalSpec  ExternalSaturationOutDataTypeStr=Inherit: Same as second input
      settings: LibrarySourceBlock=cstblocks/Linear Parameter Varying/Discrete Varying PID
  Out1 : Outport
  wires:
  Constant2/1 -> Discrete Varying PID/4
  Discrete Varying PID/1 -> Out1/1
  Constant3/1 -> Discrete Varying PID/5
  Constant/1 -> Discrete Varying PID/2
  Constant1/1 -> Discrete Varying PID/3
  In1/1 -> Discrete Varying PID/1

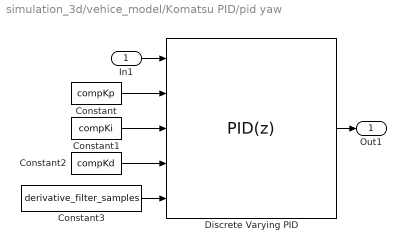
== system simulation_3d/vehice_model/Komatsu PID/pid yaw ==
  In1 : Inport
  Constant : Constant  Value=compKp
  Constant1 : Constant  Value=compKi
  Constant2 : Constant  Value=compKd
  Constant3 : Constant  Value=derivative_filter_samples
  Discrete Varying PID : slpidlib/PID Controller  Controller=PID  Form=Parallel  TimeDomain=Discrete-time  UseExternalTs=off  SampleTime=-1  IntegratorMethod=Forward Euler  FilterMethod=Forward Euler  ControllerParametersSource=external  P=1  I=1  UseKiTs=off  D=0  N=100  UseFilter=on  TunerSelectOption=Transfer Function Based (PID Tuner App)  InitialConditionSource=internal  InitialConditionForIntegrator=0  InitialConditionForFilter=0  DifferentiatorICPrevScaledInput=0  ExternalReset=none  TrackingMode=off  Kt=1  LimitOutput=off  SatLimitsSource=internal  UpperSaturationLimit=inf  LowerSaturationLimit=-inf  LinearizeAsGain=on  AntiWindupMode=none  Kb=1  LimitIntegrator=off  UpperIntegratorSaturationLimit=inf  LowerIntegratorSaturationLimit=-inf  POutMin=[]  POutMax=[]  IOutMin=[]  IOutMax=[]  DOutMin=[]  DOutMax=[]  NOutMin=[]  NOutMax=[]  SumOutMin=[]  SumOutMax=[]  SaturationOutMin=[]  SaturationOutMax=[]  PParamMin=[]  PParamMax=[]  IParamMin=[]  IParamMax=[]  DParamMin=[]  DParamMax=[]  NParamMin=[]  NParamMax=[]  KbParamMin=[]  KbParamMax=[]  KtParamMin=[]  KtParamMax=[]  KbOutMin=[]  KbOutMax=[]  KtOutMin=[]  KtOutMax=[]  IntegratorOutMin=[]  IntegratorOutMax=[]  FilterOutMin=[]  FilterOutMax=[]  SumI1OutMin=[]  SumI1OutMax=[]  SumI2OutMin=[]  SumI2OutMax=[]  SumI3OutMin=[]  SumI3OutMax=[]  SumI4OutMin=[]  SumI4OutMax=[]  SumDOutMin=[]  SumDOutMax=[]  DifferentiatorOutMin=[]  DifferentiatorOutMax=[]  FilterDiffOutCoefMin=[]  FilterDiffOutCoefMax=[]  ReciprocalOutMin=[]  ReciprocalOutMax=[]  SumDenOutMin=[]  SumDenOutMax=[]  SumNumOutMin=[]  SumNumOutMax=[]  DivideOutMin=[]  DivideOutMax=[]  UdiffTsProdOutMin=[]  UdiffTsProdOutMax=[]  NTsProdOutMin=[]  NTsProdOutMax=[]  UintegralTsProdOutMin=[]  UintegralTsProdOutMax=[]  UngainTsProdOutMin=[]  UngainTsProdOutMax=[]  ClampingZeroOutDataTypeStr=Inherit: Inherit via back propagation  ClampingZeroOutMin=[]  ClampingZeroOutMax=[]  FilterDenConstantOutDataTypeStr=Inherit: Inherit via back propagation  FilterDenConstantOutMin=[]  FilterDenConstantOutMax=[]  PCopyOutDataTypeStr=Inherit: Inherit via back propagation  PCopyOutMin=[]  PCopyOutMax=[]  NCopyOutDataTypeStr=Inherit: Inherit via back propagation  NCopyOutMin=[]  NCopyOutMax=[]  IntegratorContinuousStateAttributes=''  IntegratorStateMustResolveToSignalObject=off  IntegratorRTWStateStorageClass=Auto  FilterContinuousStateAttributes=''  FilterStateMustResolveToSignalObject=off  FilterRTWStateStorageClass=Auto  ParallelPVariant=ExternalParameters  IdealPVariant=Disabled  IVariant=ExternalParameters  DVariant=ExternalParameters  IntegratorVariant=Discrete  SatVariant=Disabled  AWVariant=Passthrough  PCopyVariant=Disabled  TRVariant=Disabled  FdbkBlocksVariant=Forward  IdealPFdbkVariant=Disabled  SatFdbkVariant=Disabled  DerivativeFilterVariant=ForwardEulerFilter  NVariant=ExternalParameters  NCopyVariant=Disabled  FilterICVariant=InternalICsFilter  IntegratorICVariant=InternalICs  ExternalResetVariant=Disabled  TRSumVariant=Passthrough  SumFdbkVariant=Disabled  SumVariant=Sum_PID  TsampFilterVariant=InternalTs  TsampNgainVariant=Passthrough  TsampIntegralVariant=Disabled_SignalSpec  ExternalSaturationOutDataTypeStr=Inherit: Same as second input
      settings: LibrarySourceBlock=cstblocks/Linear Parameter Varying/Discrete Varying PID
  Out1 : Outport
  wires:
  Constant2/1 -> Discrete Varying PID/4
  Discrete Varying PID/1 -> Out1/1
  Constant3/1 -> Discrete Varying PID/5
  Constant/1 -> Discrete Varying PID/2
  Constant1/1 -> Discrete Varying PID/3
  In1/1 -> Discrete Varying PID/1

== matlab function simulation_3d/vehice_model/vehicle_dynamics ==
  data: tau input; Rl input; Fy input; Mr input; Fb input; Mb input; q input; q_dot input; x_ICR input; x_ICR_dot input; v input; new_bld_ang input; vd_parmas input; v_dot output
function v_dot = vehicle_dynamics(tau, Rl, Fy, Mr, Fb, Mb, q, q_dot, x_ICR, x_ICR_dot, v, new_bld_ang, vd_parmas)
    % calculate and return the accleration of the vehicle from the equations of motion
    
    % unpack the body angles (roll, pitch, yaw)
    a = q(4); B = q(5); g = q(6); 
    
    % unpack the body velocities  (roll_vel, pitch_vel, yaw_vel)
    Ad = q_dot(5); Bd = q_dot(5); Gd = q_dot(6); 
    
    % unpack function parameters
    m = vd_parmas(1); h = vd_parmas(2); b = vd_parmas(3); l = vd_parmas(4); 
    r = vd_parmas(5); grav = vd_parmas(6); 

    if x_ICR == 0
        x_ICR = realmax;
    end

    sa = sin(a); ca = cos(a); sB = sin(B); cB = cos(B); sg = sin(g); cg = cos(g);
    
    ab = new_bld_ang(1); Bb = new_bld_ang(2); gb = new_bld_ang(3);
    cab = cos(ab);  sab = sin(ab); cBb = cos(Bb);  
    sBb = sin(Bb); cgb = cos(gb);  sgb = sin(gb); 

    % rotation matrix from blade to local body frame (R is orthonormal -> R^-1 = R^T)
    R_blade = [cBb*cgb, sab*sBb*cgb - cab*sgb, cab*sBb*cgb + sab*sgb;
               cBb*sgb, sab*sBb*sgb + cab*cgb, cab*sBb*sgb - sab*cgb;
                  -sBb,               sab*cBb,              cab*cBb];
    
    % moment of inertia for a plate around center
    Ix = 1/12 * m * (b^2 + h^2);
    Iy = 1/12 * m * (h^2 + l^2);
    Iz = 1/12 * m * (b^2 + l^2);
    
    % rotation matrix from local to global (R is orthonormal -> R^-1 = R^T)
    R_lg = [cB*cg, sa*sB*cg - ca*sg, ca*sB*cg + sa*sg;
            cB*sg, sa*sB*sg + ca*cg, ca*sB*sg - sa*cg;
              -sB,            sa*cB,            ca*cB];
         
    % rotation matrix from local to global of local x, y, and z
    R_lg_x = [cB*cg;
              cB*sg;
               -sB];
    R_lg_y = [sa*sB*cg - ca*sg;
            sa*sB*sg + ca*cg;
                       sa*cB];
    R_lg_z = [ca*sB*cg + sa*sg;
             ca*sB*sg - sa*cg;
                        ca*cB];

    % null space of A matrix
    S = [       R_lg_x,               R_lg_y;
         zeros([3, 1]), R_lg_z .* (-1/x_ICR)];

    % forward track forces
    B  = [    R_lg_x,    R_lg_x; 
                   0,         0; 
                   0,         0; 
          -ca*cB*b/2, ca*cB*b/2];  
     
    %resistive_forces_and_moments
    elim = [1, 0, 0, 0, 0, 0;
            0, 1, 0, 0, 0, 0;
            0, 0, 1, 0, 0, 0;
            0, 0, 0, 0, 0, 0;
            0, 0, 0, 0, 0, 0;
            0, 0, 0, 0, 0, 1];
    
    Ct = [Rl(1) + Rl(2); Fy; 0; 0; 0; Mr + (Rl(2) - Rl(1))*b/2];
    Cb = elim * [R_blade, zeros(3); zeros(3), R_blade] * [Fb; 0; 0; 0; 0; Mb];
    C = [R_lg, zeros(3); zeros(3), R_lg] * (Ct + Cb);

    % matrix relating to the mass and moment of inertia to the linear and angular kinetic energy
    M = [m, 0, 0,  0,  0,  0;
         0, m, 0,  0,  0,  0;
         0, 0, m,  0,  0,  0;
         0, 0, 0, Ix,  0,  0;
         0, 0, 0,  0, Iy,  0;
         0, 0, 0,  0,  0, Iz];
                         
    % matrix relating to the graviational potential energy
    P = [0; 0; m*grav; 0; 0; 0];

    S_11 = -sB*cg*Bd - cB*sg*Gd;
    S_21 = (ca*sB*cg + sa*sg)*Ad + sa*cB*cg*Bd - (sa*sB*sg + ca*cg)*Gd;
    S_31 = (ca*sg - sa*sB*cg)*Ad + ca*cB*cg*Bd + (sa*cg - ca*sB*sg)*Gd;
    S_12 = -sB*sg*Bd + cB*cg*Gd;
    S_22 = (ca*sB*sg - sa*cg)*Ad + sa*cB*sg*Bd + (sa*sB*cg - ca*sg)*Gd;

    S_32 = -(sa*sB*sg + ca*cg)*Ad + ca*cB*sg*Bd + (ca*sB*cg + sa*sg)*Gd;
    S_42 = cB*x_ICR^(-1)*Bd - sB*x_ICR^(-2)*x_ICR_dot;
    S_52 = -ca*cB*x_ICR^(-1)*Ad + sa*sB*x_ICR^(-1)*Bd + sa*cB*x_ICR^(-2)*x_ICR_dot;
    S_62 = sa*cB*x_ICR^(-1)*Ad + ca*sB*x_ICR^(-1)*Bd + ca*cB*x_ICR^(-2)*x_ICR_dot;
    
    Sd = [S_11, S_12;
          S_21, S_22;
          S_31, S_32;
             0, S_42;
             0, S_52;
             0, S_62];

    % tranformation of matrixes to get v_dot
    Bt = S.' * B;
    Ct = S.' * C;
    Pt = S.' * P;
    Mt = S.' * M * S;
    Et = S.' * M * Sd;

    % matrix multiplication by inverse Mt to get v_dot
    v_dot = Mt \ (Bt * tau + Ct - Et * v - Pt);
end

== matlab function simulation_3d/vehice_model/blade_and_track ==
  data: Rl output; tau input; q input; q_dot input; x_ICR input; new_bld_ang input; Fy output; Mr output; bt_params input; Fb output; Mb output
function [Rl, Fy, Mr, Fb, Mb] = blade_and_track(tau, q, q_dot, x_ICR, new_bld_ang, bt_params)
    % calculate the blade and track forces 
    
    % unpack the body angles (roll, pitch, yaw)
    a = q(4); B = q(5); g = q(6); 
    
    % unpack the body velocities and angular velocities
    X_dot = q_dot(1); Y_dot = q_dot(2); Z_dot = q_dot(3); a_dot = q_dot(4); 
    B_dot = q_dot(5); g_dot = q_dot(6);
    
    % unpack function parameters
    B1 = bt_params(1); H = bt_params(2); L = bt_params(3); b = bt_params(4); 
    l = bt_params(5); r = bt_params(6); m = bt_params(7); grav = bt_params(8); 
    velocity_limit = bt_params(9); fill_distance = bt_params(10); 
    mu_t = bt_params(11); mu_l = bt_params(12); mu_ss = bt_params(13); 
    kb = bt_params(14); gamma_g = bt_params(15); beta0 = bt_params(16); a_s = bt_params(17); 
    B_s = bt_params(18); g_s = bt_params(19); 
    
    % unpack the blade angles (roll, pitch, yaw)
    a_b = new_bld_ang(1); B_b = new_bld_ang(2); g_b = new_bld_ang(3);

    sa = sin(a); ca = cos(a); sB = sin(B); cB = cos(B); sg = sin(g); 
    cg = cos(g); 

    % calculate the cutting depth of the blade
    hp = abs(L*sin(B_b));
    
    % calculate the local forward velocity from the vehicle's global X and Y velocities
	R_gl = [cB*cg, sa*sB*cg - ca*sg, ca*sB*cg + sa*sg
        	cB*sg, sa*sB*sg + ca*cg, ca*sB*sg - sa*cg
        	  -sB,         	  sa*cB,         	ca*cB].';
   	 
	% calculate the local forward (dx) and lateral (dy) velocities
	% from the vehicle's global X and Y velocities
	dxyz = R_gl * [X_dot;Y_dot;Z_dot];
	daBg = R_gl * [a_dot;B_dot;g_dot];
    
    % Compute absolute velocities of the centre of the tracks
    vtL = dxyz(1) - b/2 * daBg(3);
    vtR = dxyz(1) + b/2 * daBg(3);
    
    vtL = saturation(vtL, velocity_limit);
    vtR = saturation(vtR, velocity_limit);
    
    % how full the pile will be out some some distance
    fill_percent = sqrt(q(1)^2+q(2)^2+q(3)^2) / fill_distance;

    [Fb, Mb] = blade_terrain_interaction(hp, kb, gamma_g, ...
                      mu_ss, a_s, beta0, a_b, B1, H, fill_percent);
    %left and right track force
    FtL = tau(1);
    FtR = tau(2);

    % longitudinal friction distribution and resistance forces
    rl  = mu_l * m*grav/2;       
    RlL = G(FtL, rl, vtL);
    RlR = G(FtR, rl, vtR);
    Rl  = [RlL; RlR];
    
    % lateral friction distribution and resistance force
    fy = mu_t * m*grav/l;
    Fy = -2 * sign(dxyz(2)) * fy * abs(x_ICR);
    
    mr = 2 * fy * ((l^2)/4 - x_ICR^2);      % resistance moment
    M  = ((FtR + RlR) - (FtL + RlL)) * b/2; % turning moment    
    Mr = G(M, mr, daBg(3));                 % moment of turning resistance
end


function [FT, Mb] = blade_terrain_interaction(hp, kb, gamma_g, ...
    mu_ss, a_s, beta0, a_b, B1, H, fill_percent)
    % calculate and return the how the ground resistants the blade

    % calcuare the relative roll of the blade to the surface and 
    % the relate soil blade heights
    a_rel = a_s - a_b;
    H1  = B1*tan(abs(a_rel));
    H2  = hp*sec(a_rel);
    H3  = H - H2 + sign(a_rel)*H1/2 - H1/2;
    H4   = H - H2 - sign(a_rel)*H1/2 - H1/2;
    
    % volume of the mound before bulldozing plate
    a = tan(abs(a_rel))^2;
    c = (H3 + H4)/2;
    V = 1/2*cot(beta0)*(1/12*a^2*B1^3 + c^2*B1);
    
    % gravity of the mound before bulldozing plate
    Gt = V * gamma_g * fill_percent;
    
    % soil-cutting resistance (N)
    hyp = B1*sec(abs(a_rel));
    area_cut = 1/2*B1*H1 + hyp*hp;
    F1 = area_cut * kb;
    
    % pushing resistance of mound before blade (N)
    F2 = Gt * mu_ss;             
    
    % blade pushback forces (N)
    FT = - F1 - F2;
    
    % calculte where the blade forces are acting
    yc1 = yc(Dx(-B1/2, beta0, H3, H4, B1), Dx(B1/2, beta0, H3, H4, B1), B1);
    yc2 = yc(H2, H1+H2, B1);
    
    % soil cutting moment acting on the blade
    Mb = yc1 * F1 + yc2 * F2;
end

== matlab function simulation_3d/vehice_model/pid (rep. hydrolics) ==
  data: bld_ang input; new_ang output; out output; ang_vel input; gain input
function [new_ang, out] = pid(bld_ang, ang_vel, gain)

    new_roll  = bld_ang(1) + gain * ang_vel(1);
    new_pitch = bld_ang(2) + gain * ang_vel(2);
    new_yaw   = bld_ang(3) + gain * ang_vel(3);
    
    new_ang = [new_roll, new_pitch, new_yaw];
    out = new_ang.';
end

== matlab function simulation_3d/vehice_model/MATLAB Function ==
  data: v input; v_sat output; v_limit input
function v_sat = vel_limiter(v, v_limit)
    v_temp = sign(v) .* min(abs(v), v_limit);
    v_sat = max(v_temp, [0;0]);
end

== matlab function simulation_3d/vehice_model/fzy_errors ==
  data: bld_ang input; depth input; errors output; des_ang input; plot output; L input; noiseless_bld_ang input
function [errors, plot] = fzy_errors(bld_ang, depth, des_ang, L, noiseless_bld_ang)
    % unpack the blade angles (roll, pitch, yaw)
    roll = bld_ang(1);          pitch = bld_ang(2);         yaw = bld_ang(3);
    nl_roll = noiseless_bld_ang(1);          nl_pitch = noiseless_bld_ang(2);         nl_yaw = noiseless_bld_ang(3);

    % unpack the desired blade angles (roll, pitch, yaw)
    desired_roll = des_ang(1); des_pitch_mult = des_ang(2); desired_yaw = des_ang(3);

    desired_pitch = des_pitch_mult * asin(depth/L);
    
    errors = [roll - desired_roll, pitch - desired_pitch, yaw - desired_yaw ];
    nl_errors = [nl_roll - desired_roll, nl_pitch - desired_pitch, nl_yaw - desired_yaw ];
    plot = [nl_errors(1), L*sin(nl_pitch), nl_errors(3)];
end

== matlab function simulation_3d/track_control_and_stopping ==
  settings: updateMethod=DISCRETE
  data: tau output; q_dot output; q output; x_ICR output; v output; bld_ang output; in input; stop output; simin input; stop_distance input
function [tau, q_dot, q, x_ICR, v, bld_ang, stop] = track_control_and_stopping(in, simin, stop_distance)
    persistent start;
    
    % initalization condition
    if isempty(start)
        in = simin;
        start = 0;
    end
    
    % bring blade angles into their controller domain, [-pi, pi]
    for i = 18:20
        if((in(i) < -pi) || (pi < in(i)))
            in(i) = mod(in(i)+pi, 2*pi) - pi;
        end
    end

    % a stop flag where nonzero values trigger the stop block
    stop = 0;
    if abs(in(9)) + abs(in(10)) > stop_distance
        stop = 1;
    end
    
    % update states
    tau     = [in(1); in(2)]; % drive wheel torques for the left and right tracks
    % an array of the global body [X_vel; Y_vel; Z_vel; roll_vel; pitch_vel; yaw_vel] 
    q_dot   = [in(3);  in(4);  in(5); in(6); in(7);   in(8)];
    % an array of the global body [X; Y; Z; roll; pitch; yaw] 
    q       = [in(9); in(10); in(11); in(12); in(13); in(14)];
    x_ICR   = in(15);                   % local body x coordinate of the Instntanous Center of Rotation  
    v       = [in(16); in(17)];         % the velocities of left and right tracks
    bld_ang = [in(18); in(19); in(20)]; %the orientation of the blade
end

== matlab function simulation_3d/vehice_model/get_x_icr ==
  data: x_ICR output; q input; q_dot input; l input
function x_ICR  = get_x_icr(q, q_dot, l)
    % get the x coordinate of the instantanous center of rotation and the
    % slip angle from the local linear and angular velocities
    
    % unpack the body angles (roll, pitch, yaw)
    a = q(4); B = q(5); g = q(6); 
    
    % unpack the body velocities and angular velocities
    X_dot = q_dot(1); Y_dot = q_dot(2); Z_dot = q_dot(3); a_dot = q_dot(4); 
    B_dot = q_dot(5); g_dot = q_dot(6); 
    
    sa = sin(a); ca = cos(a); sB = sin(B); cB = cos(B); sg = sin(g); 
    cg = cos(g);
    
    % calculate the local forward velocity from the vehicle's global X and Y velocities
	R_gl = [cB*cg, sa*sB*cg - ca*sg, ca*sB*cg + sa*sg
        	cB*sg, sa*sB*sg + ca*cg, ca*sB*sg - sa*cg
        	  -sB,         	  sa*cB,         	ca*cB].';
   	 
	% calculate the local forward (dx) and lateral (dy) velocities
	% from the vehicle's global X and Y velocities
	dxyz = R_gl * [X_dot;Y_dot;Z_dot];
	daBg = R_gl * [a_dot;B_dot;g_dot];
    
    1;

    % Avoid a divide by infinity error with the if statement
    if abs(daBg(3)) < 0.001
        x_ICR = 0;
    else
        x_ICR = dxyz(2)/daBg(3);
        x_ICR = max(-l/2, min(x_ICR, l/2));
    end
    
end

== matlab function simulation_3d/vehice_model/v_to_q_dot ==
  data: q input; x_ICR input; q_dot output; v input
function q_dot = v_to_q_dot(q, x_ICR, v)
    % calculate and return the global velocities using a transfromation from the
    % local to global frame
    
    % unpack the body angles (roll, pitch, yaw)
    a = q(4); B = q(5); g = q(6); 
    
    sa = sin(a); ca = cos(a); sB = sin(B); cB = cos(B); sg = sin(g); cg = cos(g);
    
    if abs(x_ICR) < 0.001
        x_ICR = realmax;
    end
     % rotation matrix from local to global of local x, y, and z
        R_lg_x = [cB*cg;
                  cB*sg;
                   -sB];
        R_lg_y = [sa*sB*cg - ca*sg;
                sa*sB*sg + ca*cg;
                           sa*cB];
       R_lg_z = [ca*sB*cg + sa*sg;
                 ca*sB*sg - sa*cg;
                            ca*cB];
    
        % null space of A matrix
        S = [       R_lg_x,               R_lg_y;
             zeros([3, 1]), R_lg_z .* (-1/x_ICR)];

     % the global velocities
     q_dot = S*v;
end
